simulink model "HINF"  (R2025b)
settings: Solver=ode15s  StartTime=0.0  StopTime=20  RelTol=1e-3
libraries: cstblocks x2
settings Model: Creator=salvo  LastModifiedBy=salvo

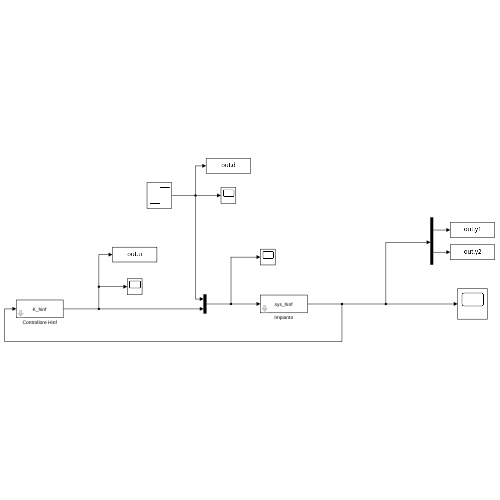
[thumbnail: Simulink's stored preview of the top-level diagram]
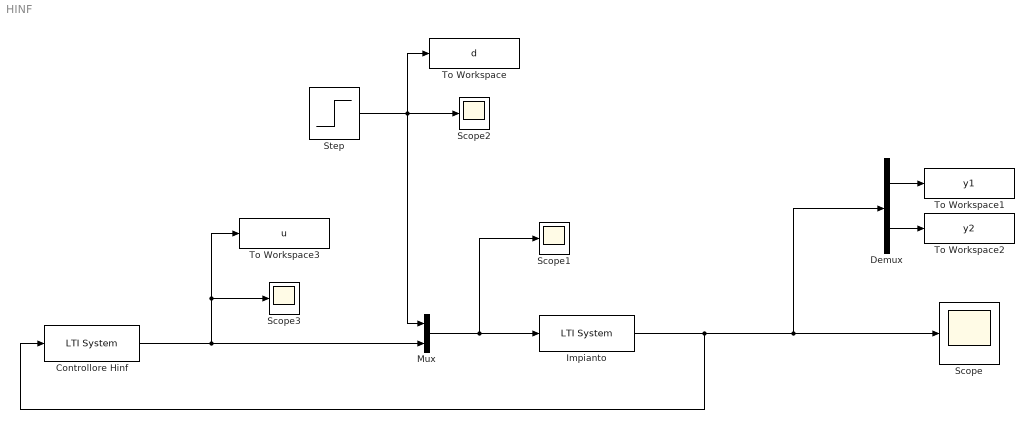
== system HINF ==
  Controllore Hinf : cstblocks/LTI System  sys=K_hinf  IC=[]  PadeOrder=0
  Demux : Demux  Outputs=2
  Impianto : cstblocks/LTI System  sys=sys_hinf  IC=[]  PadeOrder=0
  Mux : Mux  Inputs=2
  Scope{,1..3} (4 alike) : Scope
      Scope settings: ActiveDisplayYMinimum=-0.00571820347431817  ActiveDisplayYMaximum=0.0051239392725681739
      Scope1 settings: ActiveDisplayYMinimum=-1.4726435708685039  ActiveDisplayYMaximum=-0.51472962781218445
      Scope2 settings: ActiveDisplayYMinimum=-1.5137800163977375  ActiveDisplayYMaximum=4.1587693509875123  DataLoggingVariableName=ScopeData2
      Scope3 settings: ActiveDisplayYMinimum=-0.40236397787673311  ActiveDisplayYMaximum=0.084645115208972388  DataLoggingVariableName=ScopeData3
  Step : Step  Time=10  SampleTime=0
  To Workspace : ToWorkspace  VariableName=d  SaveFormat=Timeseries  SampleTime=-1
  To Workspace1 : ToWorkspace  VariableName=y1  SaveFormat=Timeseries  SampleTime=-1
  To Workspace2 : ToWorkspace  VariableName=y2  SaveFormat=Timeseries  SampleTime=-1
  To Workspace3 : ToWorkspace  VariableName=u  SaveFormat=Timeseries  SampleTime=-1
  wires:
  Mux/1 -> Scope1/1, Impianto/1
  Controllore Hinf/1 -> Mux/2, Scope3/1, To Workspace3/1
  Step/1 -> To Workspace/1, Mux/1, Scope2/1
  Impianto/1 -> Demux/1, Scope/1, Controllore Hinf/1
  Demux/1 -> To Workspace1/1
  Demux/2 -> To Workspace2/1
